simulink model "passThrough"  (R2019b)
settings: Solver=FixedStepDiscrete  StartTime=0.0  StopTime=100  RelTol=1e-3
undefined symbols (not defined in the file): xc7vx485tffg1157
libraries: ModelComposer x4, xbsIndex_r4 x2, dspsrcs4 x1
settings Model: Creator=shirazi  LastModifiedBy=abehbood
settings SFSimCC: CustomCodeUndefinedFunction=UseInterfaceOnly

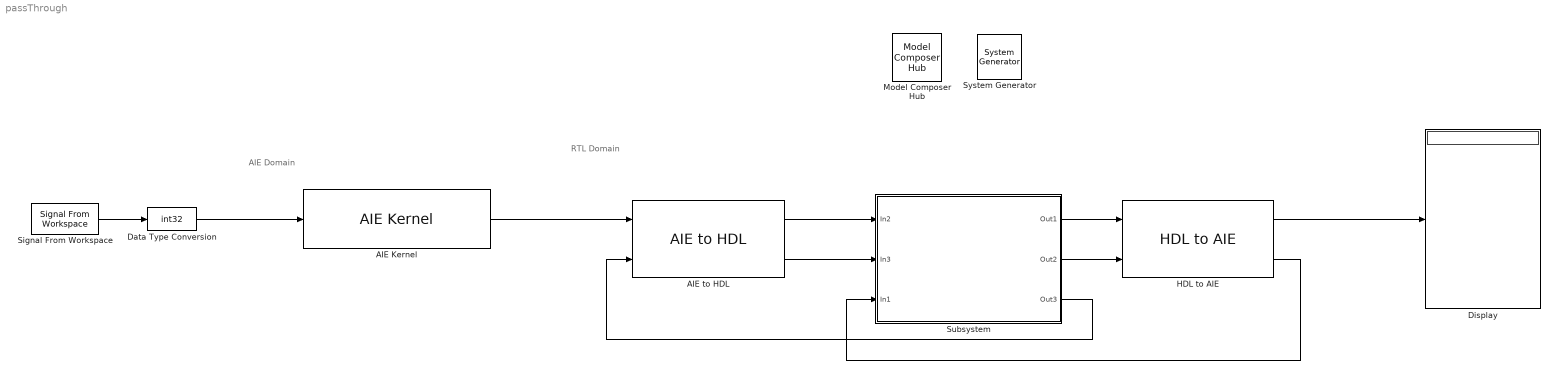
== system passThrough ==
  note: AIE Domain
  note: RTL Domain
  " System Generator" : xbsIndex_r4/ System Generator  Tag=genX  xilinxfamily=kintex7  part=xc7k325t  speed=-3  package=fbg676  synthesis_tool=Vivado  clock_wrapper=Clock Enables  directory=./netlist  proj_type=Vivado  Synth_file=Vivado Synthesis Defaults  Impl_file=Vivado Implementation Defaults  testbench=off  simulink_period=1  sysclk_period=10  dcm_input_clock_period=10  incr_netlist=off  trim_vbits=Everywhere in SubSystem  dbl_ovrd=According to Block Masks  core_generation=According to Block Masks  run_coregen=off  deprecated_control=off  eval_field=0  block_type=sysgen
  AIE Kernel : ModelComposer/AIE Kernel  PortAttributesTable={ 'Input', '_arg0', 'input_window_int32 *', '8', '0', 'sync', ''; 'Output', '_arg1', 'output_window_int32 *', '8', '', 'sync', '' }  PortAttributesEnablement={'off', 'off', 'off', 'on', 'on', 'on', 'off';'off', 'off', 'off', 'on', 'off', 'on', 'off'}  FormalArgDecls={'input_window_int32 * _arg0', 'output_window_int32 * _arg1'}  PortWindowSizes={8.000000000000000000e+00, 8.000000000000000000e+00}  PortWindowMargins={0.000000000000000000e+00, 0.000000000000000000e+00}  PortSynchronicities={'sync', 'sync'}  PortSignalSizes={0.000000000000000000e+00, 0.000000000000000000e+00}  SimLibPath=''  FunctionTabVisible=on  FunctionDescription=void mysquare(input_window_int32 * _arg0, output_window_int32 * _arg1)  KernelHeaderFile=mysquare.h  KernelFunction=mysquare  KernelFunctionSelect=<empty>  KernelSourceFile=mysquare.cc  KernelSearchPaths={}  PreProcOptions={}  CoreRuntimeRatio=0.9
  AIE to HDL : ModelComposer/AIE to HDL  OutDataType=int32  OutSampleTime=1
  Data Type Conversion : DataTypeConversion  OutDataTypeStr=int32
  Display : Display
  HDL to AIE : ModelComposer/HDL to AIE  OutDataType=int32  OutSampleTime=1  SamplesPerFrame=8  TreadySampleTime=1
  Model Composer Hub : ModelComposer/Model Composer Hub  CodeGeneration=off  TargetDirectory=./aie_code  SubsystemName=AIE_Subsystem  ExportType=AI Engines  IpVendor=xilinx.com  IpLibrary=hls  IpVersion=1.0  IpHWLanguage=Verilog  CreateTestbench=off  TestbenchStackSize=10  AieCompilerOptions={}  RunAieSim=off  LaunchVitisAnalyzer=off  AieSimTimeout=50000  RunX86Sim=on  X86SimTimeout=10  ProjDevice=xc7vx485tffg1157-1  ProjDevicePart=xc7vx485tffg1157-1  SamplePeriod=-1  ClockFrequency=200  DataPathParallelism=1
  Signal From Workspace : dspsrcs4/Signal From Workspace  X=1:100  Ts=1  nsamps=8  OutputAfterFinalValue=Cyclic repetition  ignoreOrWarnInputAndFrameLengths=off  OutputFrames=off
  Subsystem : Subsystem
  wires:
  Signal From Workspace/1 -> Data Type Conversion/1
  Data Type Conversion/1 -> AIE Kernel/1
  HDL to AIE/1 -> Display/1
  Subsystem/1(Out1) -> HDL to AIE/1
  AIE to HDL/1 -> Subsystem/1(In2)
  Subsystem/2(Out2) -> HDL to AIE/2
  AIE Kernel/1 -> AIE to HDL/1
  AIE to HDL/2 -> Subsystem/2(In3)
  HDL to AIE/2 -> Subsystem/3(In1)
  Subsystem/3(Out3) -> AIE to HDL/2

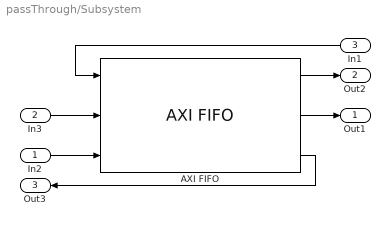
== system passThrough/Subsystem ==
  In2 : Inport
  In3 : Inport  Port=2
  In1 : Inport  Port=3
  AXI FIFO : xbsIndex_r4/AXI FIFO  input_depth_axis=1K  actual_fifo_depth_label=1026  enable_tdata=on  enable_tdest=off  enable_tstrb=off  enable_tready=on  enable_tid=off  enable_tuser=off  enable_tkeep=off  enable_tlast=off  has_aresetn=off  enable_data_counts_axis=off  fifo_implementation_type_axis=Common Clock Block RAM  trim_axipin_name=off  programmable_full_type_axis=Full  full_threshold_assert_value_axis=0  programmable_empty_type_axis=Empty  empty_threshold_assert_value_axis=1022  underflow_flag_axi=0  underflow_sense_axi=Active High  overflow_flag_axi=0  overflow_sense_axi=Active High  simulation_type=fast_sim  block_type=axi_fifo
  Out1 : Outport
  Out2 : Outport  Port=2
  Out3 : Outport  Port=3
  wires:
  AXI FIFO/2 -> Out1/1
  AXI FIFO/1 -> Out2/1
  In1/1 -> AXI FIFO/1
  AXI FIFO/3 -> Out3/1
  In2/1 -> AXI FIFO/3
  In3/1 -> AXI FIFO/2
